simulink model "Vozmushenie"  (R2017a)
settings: Solver=VariableStepAuto  StartTime=0.0  StopTime=30  RelTol=1e-6
settings Model: Creator=User  LastModifiedBy=User

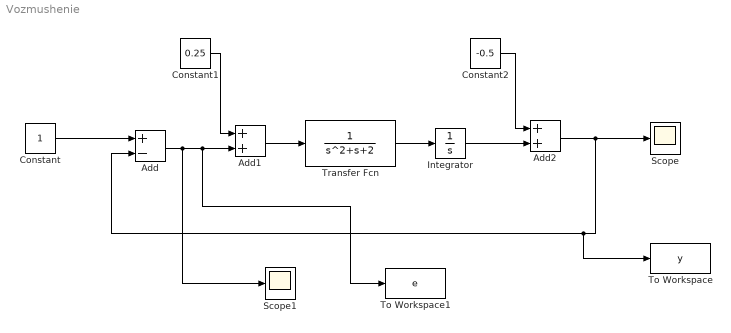
== system Vozmushenie ==
  Add : Sum  Inputs=+-
  Add1 : Sum
  Add2 : Sum
  Constant : Constant
  Constant1 : Constant  Value=0.25
  Constant2 : Constant  Value=-0.5
  Integrator : Integrator
  Scope : Scope
  Scope1 : Scope
  To Workspace : ToWorkspace  VariableName=y  SampleTime=-1
  To Workspace1 : ToWorkspace  VariableName=e  SampleTime=-1
  Transfer Fcn : TransferFcn  Denominator=[1 1 2]
  wires:
  Add/1 -> To Workspace1/1, Add1/2, Scope1/1
  Transfer Fcn/1 -> Integrator/1
  Constant/1 -> Add/1
  Add1/1 -> Transfer Fcn/1
  Integrator/1 -> Add2/2
  Add2/1 -> To Workspace/1, Add/2, Scope/1
  Constant1/1 -> Add1/1
  Constant2/1 -> Add2/1
